simulink model "az_first"  (R2020b)
settings: Solver=ode45  StartTime=0.0  StopTime=50  RelTol=1e-3  EnableMultiTasking=on
Description:
  | Simulating Automatic Climate Control Systems
  | 
  | This example shows how to use Simulink(R) and Stateflow(R) to simulate the working of
  | an automatic climate control system in a car. You can enter a temperature
  | value you would like the air in the car to reach by double clicking the
  | User Setpoint in Celsius Block and entering the temperature value. You can
  | also set the External Temperature in Celsius in a similar way. The
  | numerical display on the right-hand side of the model shows the reading
  | of a temperature sensor placed behind the driver's head. This is the
  | temperature that the driver should be feeling. When the model is run and
  | the climate control is active, it is this display box whose value changes
  | to show the change of temperature in the car.
settings Model: FPTRunName=Active  ExtModeAutoUpdateStatusClock=off  Creator=The MathWorks, Inc.  LastModifiedBy=admin
settings DataIOCC: LimitDataPoints=on  SaveFormat=Array  ReturnWorkspaceOutputs=off  SignalLoggingName=sigsOut
settings OptimizationCC: ExpressionDepthLimit=2147483647  InitFltsAndDblsToZero=on  LifeSpan=inf
settings DebuggingCC: SaveWithParameterizedLinksMsg=none  SignalResolutionControl=TryResolveAllWithWarning  MultiTaskDSMMsg=warning  MultiTaskCondExecSysMsg=none  SigSpecEnsureSampleTimeMsg=none  FcnCallInpInsideContextMsg=warning  StateNameClashWarn=warning  SFUnexpectedBacktrackingDiag=warning  SFNoUnconditionalDefaultTransitionDiag=warning  SFExecutionAtInitializationDiag=none  ArithmeticOperatorsInVariantConditions=warning
settings HardwareCC: ProdBitPerPointer=32  ProdBitPerSizeT=32  ProdBitPerPtrDiffT=32  ProdLargestAtomicFloat=None  ProdIntDivRoundTo=Undefined  ProdEndianess=Unspecified  ProdWordSize=32  ProdHWDeviceType=32-bit Generic
settings ModelReferenceCC: PropagateSignalLabelsOutOfModel=off
settings SFSimCC: SimUseLocalCustomCode=off  SimParseCustomCode=off  CustomCodeUndefinedFunction=UseInterfaceOnly
settings RTWCC: RTWUseLocalCustomCode=off
settings CodeAppCC: StateflowObjectComments=on
settings GRTTargetCC: TargetFcnLib=ansi_tfl_tmw.mat  TargetLangStandard=C89/C90 (ANSI)  CombineOutputUpdateFcns=off  GRTInterface=on
settings ConfigComp: CovMetricSettings=dw  CovSaveCumulativeToWorkspaceVar=on  CovSaveSingleToWorkspaceVar=on  CovExternalEMLEnable=off  CovSFcnEnable=off

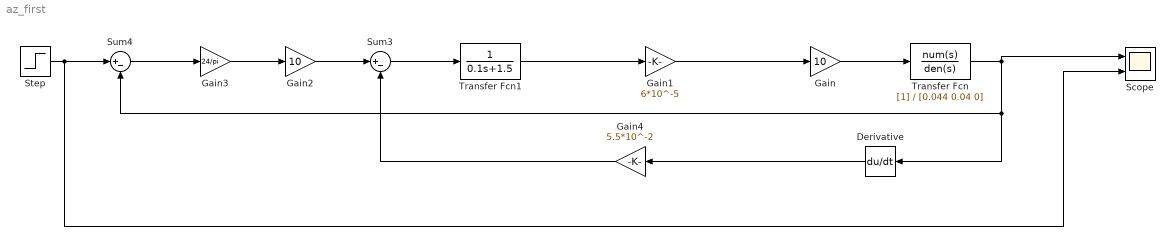
== system az_first ==
  Derivative : Derivative
  Gain : Gain  Gain=10
  Gain1 : Gain  Gain=6*10^-5
  Gain2 : Gain  Gain=10
  Gain3 : Gain  Gain=24/pi
  Gain4 : Gain  Gain=5.5*10^-2
  Scope : Scope  NumInputPorts=2
  Step : Step  SampleTime=0
  Sum3 : Sum  Inputs=|+-
  Sum4 : Sum  Inputs=|+-
  Transfer Fcn : TransferFcn  Denominator=[0.044 0.04 0]
  Transfer Fcn1 : TransferFcn  Denominator=[0.1 1.5]
  wires:
  Transfer Fcn/1 -> Sum4/2, Derivative/1, Scope/1
  Derivative/1 -> Gain4/1
  Transfer Fcn1/1 -> Gain1/1
  Gain1/1 -> Gain/1
  Gain/1 -> Transfer Fcn/1
  Sum3/1 -> Transfer Fcn1/1
  Step/1 -> Scope/2, Sum4/1
  Sum4/1 -> Gain3/1
  Gain3/1 -> Gain2/1
  Gain4/1 -> Sum3/2
  Gain2/1 -> Sum3/1
